simulink model "tf_rc_xc"  (R2016a)
settings: Solver=VariableStepAuto  StartTime=0.0  StopTime=10.0  RelTol=1e-3
values from neighbouring files (symbols this model uses):
  B_ar = [1 0 0 0 0]'    [main.m]
  B_au = [0 0 0 440 0]'    [main.m]
  c = 3.5e-2    (= 0.035)    [main.m]
  k = 42    [main.m]    (also in test_usw.m = [3,0.1])
  k_ac = 51    [main.m]
  k_af = 2.59e-2    (= 0.0259)    [main.m]
  m_c = 8.5    [main.m]
  m_f = 0.7e-3    (= 0.0007)    [main.m]
  S = [-1.7e6 2.28e4 225 1.91 2.71]    [main.m]
undefined symbols (not defined in the file or in its folder): A_a, A_lpf, B_lpf, C_lpf, k_sigm, k_sw1, k_sw2
settings Model: Creator=chao  LastModifiedBy=chao

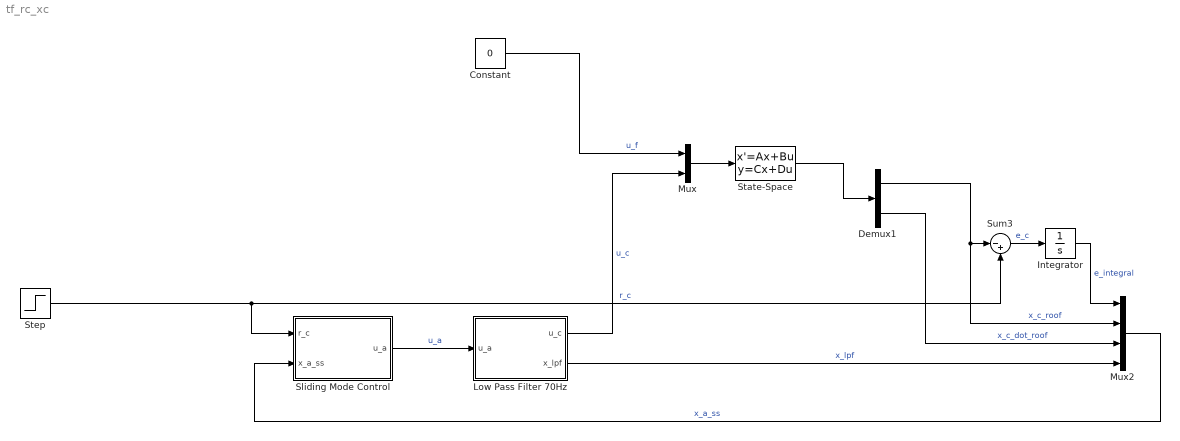
== system tf_rc_xc ==
  Constant : Constant  Value=0
  Demux1 : Demux  Outputs=2
  Integrator : Integrator
  Low Pass Filter 70Hz : Subsystem
  Mux : Mux  Inputs=2
  Mux2 : Mux
  Sliding Mode Control : Subsystem
  State-Space : StateSpace  A=[0, 1, 0, 0; -k/m_f, -c/m_f, k/m_f, c/m_f;0, 0, 0, 1; 0, 0, 0, 0]  B=[0, 0; k_af/m_f, 0;0, 0; 0, k_ac/m_c];  C=[0 0 1 0;0 0 0 1]  D=[0 0;0 0]  X0=0
  Step : Step  SampleTime=0
  Sum3 : Sum  Inputs=|-+
  wires:
  Constant/1 -> Mux/1  "u_f"
  Mux/1 -> State-Space/1
  Sum3/1 -> Integrator/1  "e_c"
  State-Space/1 -> Demux1/1
  Demux1/1 -> Mux2/2, Sum3/1  "x_c_roof"
  Integrator/1 -> Mux2/1  "e_integral"
  Demux1/2 -> Mux2/3  "x_c_dot_roof"
  Low Pass Filter 70Hz/1(u_c) -> Mux/2  "u_c"
  Mux2/1 -> Sliding Mode Control/2(x_a_ss)  "x_a_ss"
  Sliding Mode Control/1(u_a) -> Low Pass Filter 70Hz/1(u_a)  "u_a"
  Low Pass Filter 70Hz/2(x_lpf) -> Mux2/4  "x_lpf"
  Step/1 -> Sliding Mode Control/1(r_c), Sum3/2  "r_c"

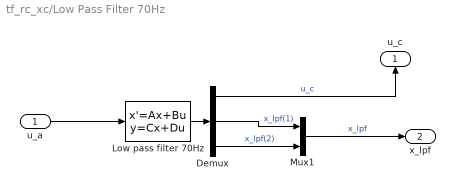
== system tf_rc_xc/Low Pass Filter 70Hz ==
  u_a : Inport
  Demux : Demux  Outputs=3
  Low pass filter 70Hz : StateSpace  A=A_lpf  B=B_lpf  C=[C_lpf;1 0;0 1]  D=[0;0;0]  X0=0
  Mux1 : Mux  Description=x_lpf  Inputs=2
  u_c : Outport
  x_lpf : Outport  Port=2
  wires:
  Demux/3 -> Mux1/2  "x_lpf(2)"
  Demux/1 -> u_c/1  "u_c"
  Low pass filter 70Hz/1 -> Demux/1
  Mux1/1 -> x_lpf/1  "x_lpf"
  Demux/2 -> Mux1/1  "x_lpf(1)"
  u_a/1 -> Low pass filter 70Hz/1

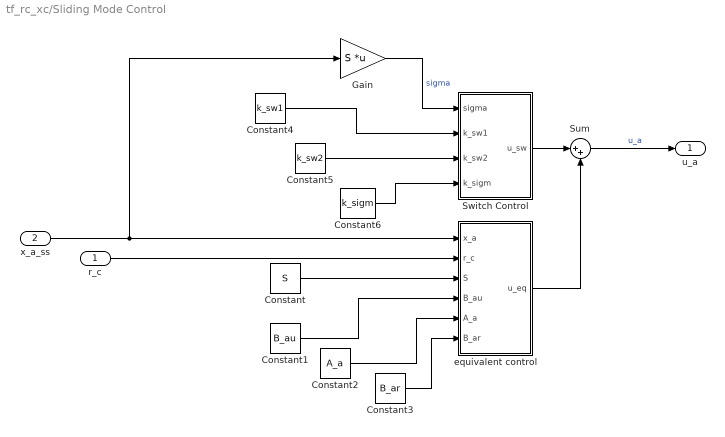
== system tf_rc_xc/Sliding Mode Control ==
  r_c : Inport
  x_a_ss : Inport  Port=2
  Constant : Constant  Value=S  VectorParams1D=off
  Constant1 : Constant  Value=B_au  VectorParams1D=off
  Constant2 : Constant  Value=A_a  VectorParams1D=off
  Constant3 : Constant  Value=B_ar  VectorParams1D=off
  Constant4 : Constant  Value=k_sw1
  Constant5 : Constant  Value=k_sw2
  Constant6 : Constant  Value=k_sigm
  Gain : Gain  Gain=S  Multiplication=Matrix(K*u)
  Sum : Sum  Inputs=|++
  Switch Control : MATLAB Function  TreatAsAtomicUnit=on
  equivalent control : MATLAB Function  TreatAsAtomicUnit=on
  u_a : Outport
  wires:
  r_c/1 -> equivalent control/2(r_c)
  Switch Control/1(u_sw) -> Sum/1
  equivalent control/1(u_eq) -> Sum/2
  Sum/1 -> u_a/1  "u_a"
  Gain/1 -> Switch Control/1(sigma)  "sigma"
  x_a_ss/1 -> equivalent control/1(x_a), Gain/1
  Constant/1 -> equivalent control/3(S)
  Constant3/1 -> equivalent control/6(B_ar)
  Constant2/1 -> equivalent control/5(A_a)
  Constant1/1 -> equivalent control/4(B_au)
  Constant4/1 -> Switch Control/2(k_sw1)
  Constant5/1 -> Switch Control/3(k_sw2)
  Constant6/1 -> Switch Control/4(k_sigm)

== matlab function tf_rc_xc/Sliding Mode Control/Switch Control ==
  data: sigma input; u_sw output; k_sw1 input; k_sw2 input; k_sigm input
function u_sw = fcn(sigma, k_sw1, k_sw2, k_sigm)

u_sw = (-k_sw1*sign(sigma)-k_sw2*sigma).*abs(2./(1+exp(-k_sigm*sigma))-1);

== matlab function tf_rc_xc/Sliding Mode Control/equivalent control ==
  data: x_a input; u_eq output; r_c input; S input; B_au input; A_a input; B_ar input
function u_eq = fcn(x_a, r_c, S, B_au, A_a, B_ar)

u_eq = -(S*B_au)\(S*A_a*x_a+S*B_ar*r_c);
